simulink model "mDiffWheelSet"  (R2019b)
settings: configuration reference "ConfigSetDesktopVariableStep" (kept outside this file)
values from neighbouring files (symbols this model uses):
  TestVehMassFactor = 0.5    [DdTestWheels.sldd]
undefined symbols (not defined in the file or in its folder): ChassisVehMass, EnvGravCnst
libraries: LibWheels x1
settings Model: DataDictionary=DdTestWheels.sldd  EnableAccessToBaseWorkspace=off  SimulationMode=accelerator  Creator=9bt  LastModifiedBy=4qz
settings ConfigSetRef: SourceName=ConfigSetDesktopVariableStep

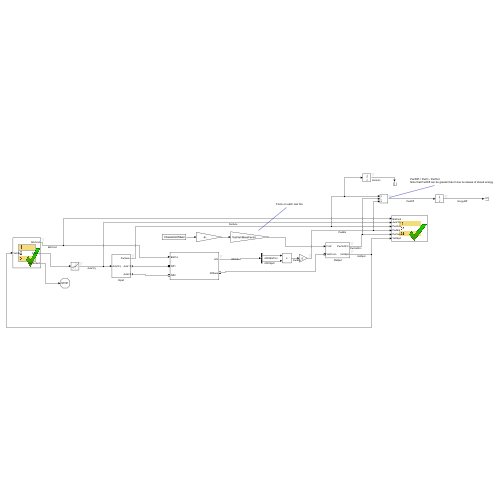
[thumbnail: Simulink's stored preview of the top-level diagram]
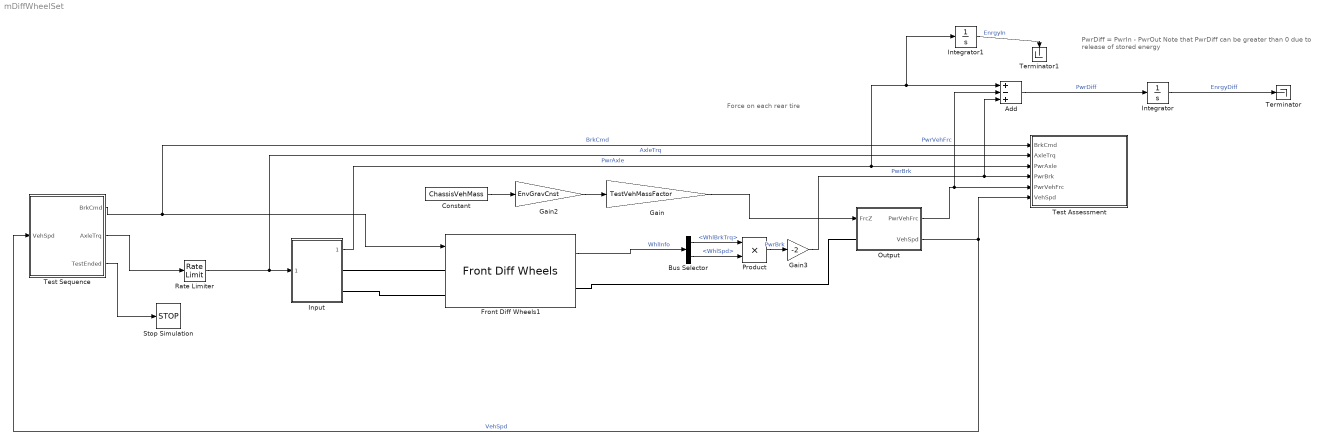
== system mDiffWheelSet ==
  note: PwrDiff = PwrIn - PwrOut
      | Note that PwrDiff can be greater than 0 due to release of stored energy
  note: Force on each rear tire
  Add : Sum  Inputs=+-+
  Bus Selector : BusSelector  OutputSignals=WhlBrkTrq,WhlSpd
  Constant : Constant  Value=ChassisVehMass
  Front Diff Wheels1 : LibWheels/Longitudinal Wheels and Brakes/Front Diff Wheels  SystemSampleTime=-1  Latency=0  AutoFrameSizeCalculation=off
  Gain : Gain  Gain=TestVehMassFactor
  Gain2 : Gain  Gain=EnvGravCnst
  Gain3 : Gain  Gain=-2
  Input : Subsystem
  Integrator : Integrator
  Integrator1 : Integrator
  Output : Subsystem
  Product : Product
  Rate Limiter : RateLimiter  RisingSlewLimit=3000  FallingSlewLimit=-3000  SampleTimeMode=inherited
  Stop Simulation : Stop
  Terminator : Terminator
  Terminator1 : Terminator
  Test Assessment : Test Sequence  TreatAsAtomicUnit=on
  Test Sequence : Test Sequence  TreatAsAtomicUnit=on
  wires:
  Test Sequence/1(BrkCmd) -> Front Diff Wheels1/1, Test Assessment/1(BrkCmd)  "BrkCmd"
  Front Diff Wheels1/1 -> Bus Selector/1  "WhlInfo"
  Test Sequence/2(AxleTrq) -> Rate Limiter/1
  Constant/1 -> Gain2/1
  Gain/1 -> Output/1(FrcZ)
  Input/1(PwrAxle) -> Integrator1/1, Add/1, Test Assessment/3(PwrAxle)  "PwrAxle"
  Output/1(PwrVehFrc) -> Test Assessment/5(PwrVehFrc), Add/2  "PwrVehFrc"
  Rate Limiter/1 -> Test Assessment/2(AxleTrq), Input/1(AxleTrq)  "AxleTrq"
  Output/2(VehSpd) -> Test Sequence/1(VehSpd), Test Assessment/6(VehSpd)  "VehSpd"
  Gain2/1 -> Gain/1
  Test Sequence/3(TestEnded) -> Stop Simulation/1
  Bus Selector/1 -> Product/1  "<WhlBrkTrq>"
  Bus Selector/2 -> Product/2  "<WhlSpd>"
  Gain3/1 -> Add/3, Test Assessment/4(PwrBrk)  "PwrBrk"
  Add/1 -> Integrator/1  "PwrDiff"
  Product/1 -> Gain3/1  "PwrBrk"
  Integrator/1 -> Terminator/1  "EnrgyDiff"
  Integrator1/1 -> Terminator1/1  "EnrgyIn"
  connections:
  Input/RConn1 -- Front Diff Wheels1/LConn1
  Input/RConn2 -- Front Diff Wheels1/LConn2
  Output/LConn1 -- Front Diff Wheels1/RConn1

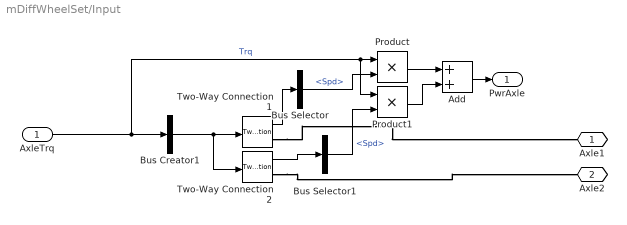
== system mDiffWheelSet/Input ==
  AxleTrq : Inport
  Add : Sum
  Bus Creator1 : BusCreator  Inputs=1
  Bus Selector : BusSelector  OutputSignals=Spd
  Bus Selector1 : BusSelector  OutputSignals=Spd
  Product : Product
  Product1 : Product
  Two-Way Connection1 : TwoWayConnection
  Two-Way Connection2 : TwoWayConnection
  Axle1 : PMIOPort  Side=Right
  Axle2 : PMIOPort  Port=2  Side=Right
  PwrAxle : Outport
  wires:
  Product1/1 -> Add/2
  AxleTrq/1 -> Product1/1, Product/1, Bus Creator1/1  "Trq"
  Product/1 -> Add/1
  Bus Creator1/1 -> Two-Way Connection2/1, Two-Way Connection1/1
  Bus Selector1/1 -> Product1/2  "<Spd>"
  Two-Way Connection1/1 -> Bus Selector/1
  Bus Selector/1 -> Product/2  "<Spd>"
  Add/1 -> PwrAxle/1
  Two-Way Connection2/1 -> Bus Selector1/1
  connections:
  Two-Way Connection1/RConn1 -- Axle1/RConn1
  Two-Way Connection2/RConn1 -- Axle2/RConn1

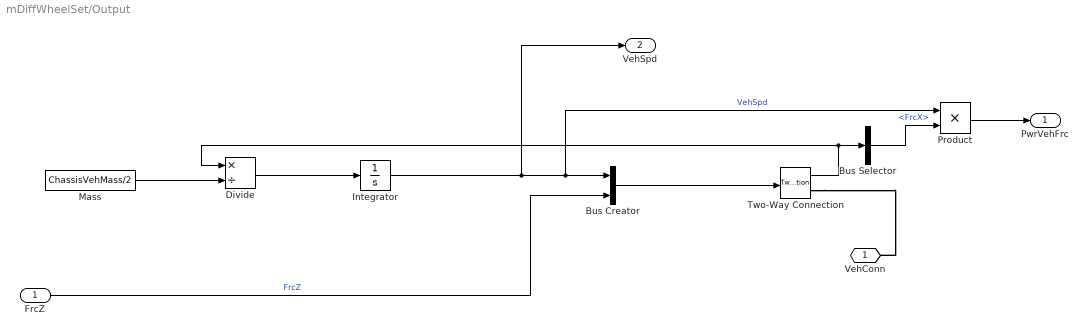
== system mDiffWheelSet/Output ==
  FrcZ : Inport
  Bus Creator : BusCreator  Inputs=2
  Bus Selector : BusSelector  OutputSignals=FrcX
  Divide : Product  Inputs=*/
  Integrator : Integrator
  Mass : Constant  Value=ChassisVehMass/2
  Product : Product
  Two-Way Connection : TwoWayConnection
  VehConn : PMIOPort  Side=Left
  PwrVehFrc : Outport
  VehSpd : Outport  Port=2
  wires:
  Bus Creator/1 -> Two-Way Connection/1
  Integrator/1 -> VehSpd/1, Product/1, Bus Creator/1  "VehSpd"
  Two-Way Connection/1 -> Divide/1, Bus Selector/1
  FrcZ/1 -> Bus Creator/2  "FrcZ"
  Bus Selector/1 -> Product/2  "<FrcX>"
  Product/1 -> PwrVehFrc/1
  Divide/1 -> Integrator/1
  Mass/1 -> Divide/2
  connections:
  Two-Way Connection/RConn1 -- VehConn/RConn1

== stateflow chart mDiffWheelSet/Test Assessment ==
  settings: stateMachineType=SIMPLIFIED_MACHINE
  state PowerCheck
    state VerifyInOutPower
      settings: description=Verify that power input to the axle is greater than the power applied to the vehicle body
    state PowerCheck_1
    PowerCheck -> (junction 22)
    (default) -> (junction 22)
    (junction 22) -> (junction 23) [order 1] : [BrkCmd == 0 && abs(VehSpd) > 2 && abs(AxleTrq) > 100
        | ]
    (junction 23) -> VerifyInOutPower [order 1] : [~in(PowerCheck.VerifyInOutPower)]
    (junction 23) -> (junction 26) [order 2]
    (junction 53) -> (junction 54)
    (junction 54) -> PowerCheck_1 [order 1] : [~in(PowerCheck.PowerCheck_1)]
    (junction 54) -> (junction 57) [order 2]
    (junction 22) -> (junction 53) [order 2]
  (default) -> PowerCheck
  data: BrkCmd input; AxleTrq input; PwrAxle input; PwrBrk input; PwrVehFrc input; VehSpd input

== stateflow chart mDiffWheelSet/Test Sequence ==
  settings: stateMachineType=SIMPLIFIED_MACHINE
  state Init
    AxleTrq = 200;
    BrkCmd = 0;
    TestEnded = false;
  state StairStepTrqUp
    state IncreaseTrq
      AxleTrq = AxleTrq + 100;
    state Wait
    (default) -> IncreaseTrq
    StairStepTrqUp.Wait -> IncreaseTrq : [
        | after(1,sec)
        | ]
    IncreaseTrq -> StairStepTrqUp.Wait : [
        | true
        | ]
  state StartCoast
    AxleTrq = 0;
    EndBrakingTest = false;
  state BrakingTest
    AxleTrq = 0;
    BrkCmd = 0.7;
    state Wait
    state VerifyForwardBraking
      verify(VehSpd < .2);
      EndBrakingTest = true;
    (default) -> BrakingTest.Wait
    BrakingTest.Wait -> VerifyForwardBraking : [
        | after(30,sec)
        | ]
  state StairStepTrqDown
    BrkCmd = 0;
    settings: description=Decrease torque to go in reverse.
    state DecreaseTrq
      AxleTrq = AxleTrq - 50;
    state Wait
    (default) -> DecreaseTrq
    DecreaseTrq -> StairStepTrqDown.Wait
    StairStepTrqDown.Wait -> DecreaseTrq : [
        | after(1, sec)
        | ]
  state StartCoast2
    AxleTrq = 0;
    EndBrakingTest = false;
  state BrakingInReverse
    AxleTrq = 0;
    BrkCmd = .7;
    state Wait
    state VerifyReverseBraking
      verify(VehSpd < .2);
      EndBrakingTest = true;
    (default) -> BrakingInReverse.Wait
    BrakingInReverse.Wait -> VerifyReverseBraking : [
        | after(10,sec)
        | ]
  state StopTrq
    AxleTrq = 0;
    BrkCmd = 0;
    TestEnded = true;
  (default) -> Init
  Init -> StairStepTrqUp : [
      | true
      | ]
  StairStepTrqUp -> StartCoast : [
      | VehSpd >= 25
      | ]
  StartCoast -> BrakingTest : [
      | after(5,sec)
      | ]
  BrakingTest -> StairStepTrqDown : [
      | EndBrakingTest == true
      | ]
  StairStepTrqDown -> StartCoast2 : [
      | VehSpd < -5
      | ]
  StartCoast2 -> BrakingInReverse : [
      | after(2,sec)
      | ]
  BrakingInReverse -> StopTrq : [
      | EndBrakingTest == true
      | ]
  data: BrkCmd output; AxleTrq output; VehSpd input; EndBrakingTest local; TestEnded output
